simulink library "SignalGeneratorLibBtc"  (R2022b)
settings: Solver=VariableStepAuto  StartTime=0.0  StopTime=10.0  RelTol=1e-3
libraries: simulink x16, FeaturePath x6, HandyTextFile x6, RTC x6, TuneVar x1
(part 1 of 2)
settings Model: Creator=yp1048186  LastModifiedBy=kl13806
settings SolverCC: AlgebraicLoopSolver=TrustRegion
settings DebuggingCC: UnconnectedInputMsg=warning  UnconnectedOutputMsg=warning  UnconnectedLineMsg=warning  SFMachineParentedDataDiag=warning
settings ModelReferenceCC: EnableRefExpFcnMdlSchedulingChecks=on
settings RTWCC: DLArmComputeVersion=19.05

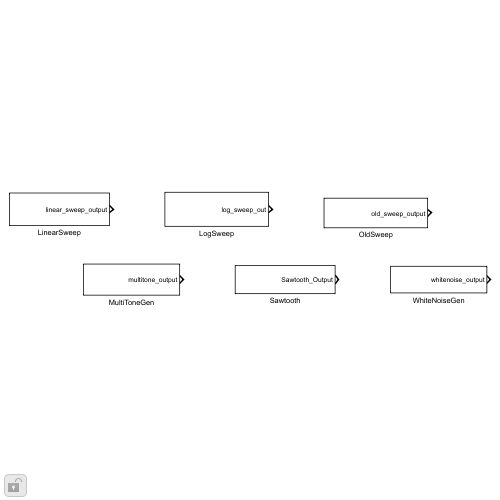
[thumbnail: Simulink's stored preview of the top-level diagram]
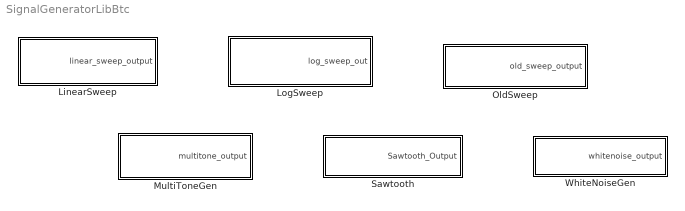
== system SignalGeneratorLibBtc ==
  LinearSweep : Subsystem  mask(Blocklib LinearSweep){Config=[], FeatureName=SignalGeneratorLinearSweep}
      mask prompts: Config "LinearSweepConfig"; FeatureName "Feature path name:"
      mask init:
      | blkh=gcbh;
      | Config=BTConfig.Assert(blkh,Config);
      | 
      | Config.Validate();
      | BTConfig.InitSetFeatureIfPresent(blkh,'FeatureName');
      mask Callback Config: BTConfig.CallbackHideIfPresent(gcbh,{'FeatureName'});
      mask TypeOptions FeatureName: FeaturePath/FeatureName
  LogSweep : Subsystem  mask(Blocklib LogSweep){Config=[], FeatureName=SignalGeneratorLogSweep}
      mask prompts: Config "LogSweepConfig"; FeatureName "Feature path name:"
      mask init:
      | blkh=gcbh;
      | Config=BTConfig.Assert(blkh,Config);
      | 
      | Config.Validate();
      | BTConfig.InitSetFeatureIfPresent(blkh,'FeatureName');
      mask Callback Config: BTConfig.CallbackHideIfPresent(gcbh,{'FeatureName'});
      mask TypeOptions FeatureName: FeaturePath/FeatureName
  MultiToneGen : Subsystem  mask(Blocklib MultiToneGen){Config=[], FeatureName=SignalGeneratorMultitone}
      mask prompts: Config "MultiToneGenConfig"; FeatureName "Feature path name:"
      mask help:
      | This block is used for generating a multi channel multi tone signal by using a sinusoid generator that supports arbirtrary frequencies by interpolating from a sine table.
      |
      | multitone_ON   :
      | Mode selection for enable/disable of multitone signal
      | 0 = Off
      | 6 = Multitone Signal
      | Example : multitone_ON =6 enables multi tone signal, multitone_ON=0 disables the multi tone signal
      |
      | multitone_channel_map   :
      | Number of tones in each channel
      | Example : multitone_channel_map = [2 3] , Indicates that there are 5 tones which needs to be mapped to 2 output channels.
      | 1st output channel has 2 tones summed up and 2nd output channel has 3 tones summed up.
      |
      | Num_Multitone_channels :
      | Indicates that there are multiple output channels ,each channel has multitone signal.
      | Example : Num_Multitone_channels=1 and multitone_channel_map =[4] means there is 1 output channel having 4 tones summed up.
      |
      | NumTones :
      | Total Number of tones
      | Example : NumTones=4 and multitone_channel_map =[4] indicates there is 1 output channel having  4 tones summed up.
      |
      | Tone_freq_Hz :
      | Vector of Frequency values in Hz for each Tone
      | Example : Tone_freq_Hz=[100 200 300]  means there are 3 tones of 100 ,200 and 300 Hz which may be assigned to 1 output channel or multiple channels
      | based on multitone_channel_map.
      | If multitone_channel_map=[1 2],this means 1st output channel will have only 100 Hz output i.e single tone signal.
      | and 2nd output channel will have 200 Hz and 300 Hz tones summed up.
      |
      | start_phase_rad :
      | Vector of Starting phase values in radians for each tone
      | Example : start_phase_rad=[0 pi/2 pi]
      |
      | ToneGains :
      | Vector of Gain values for each tone
      | Example : start_phase_rad=[0 0.25 0.5], multitone_channel_map=[3] means there is 1 output channel with 3 tones summed up and total gain observed
      | at output channel will be a sum close to 0.75
      mask init:
      | blkh=gcbh;
      | Config=BTConfig.Assert(blkh,Config);
      | 
      | Config.Validate();
      | BTConfig.InitSetFeatureIfPresent(blkh,'FeatureName');
      mask Help:
      | Configuration Parameters:
      | 
      |   multitone_ON
      |                         : mode: Vector of modes for each channel's operation
      | 						  0 = Off
      | 						  1 = Logarithmic sine sweep
      | 						  2 = Linear sine sweep
      | 						  3 = Old style sine sweep
      | 						  4 = Random noise
      | 						  5 = Sawtooth wave (Does not support sweep)
      | 						  6 = Multitone Signal
      | 						 Example : multitone_ON =6
      | 
      |   multitone_channel_map
      |                         : Number of tones in each channel
      | 						Example : multitone_channel_map = [2 3] , Indicates that there are 5 tones which needs to be mapped to 2 output channels.
      | 						1st output channel has 2 tones summed up and 2nd output channel has 3 tones summed up.
      |   Num_Multitone_channels
      |                         : Indicates that there are multiple output channels ,each channel has multitone signal.
      | 						Example : Num_Multitone_channels=1 and multitone_channel_map =[4] means there is 1 output channel having 4 tones summed up.
      |   NumTones
      |                         : Total Number of tones
      | 						Example : NumTones=4 and multitone_channel_map =[4] indicates there is 1 output channel having  4 tones summed up.
      |   Tone_freq_Hz
      |                         : Vector of Frequency values in Hz for each Tone
      | 						Example : Tone_freq_Hz=[100 200 300]  means there are 3 tones of 100 ,200 and 300 Hz which may be assigned to 1 output channel or multiple channels
      | 						based on multitone_channel_map.
      | 						If multitone_channel_map=[1 2],
      | 						this means 1st output channel will have only 100 Hz output i.e single tone signal.
      | 						and 2nd output channel will have 200 Hz and 300 Hz tones summed up.
      |   start_phase_rad
      |                         : Vector of Starting phase values in radians for each tone
      | 						Example : start_phase_rad=[0 pi/2 pi]
      |   ToneGains
      |                         : Vector of Gain values for each tone
      | 						Example : start_phase_rad=[0 0.25 0.5], multitone_channel_map=[3] means there is 1 output channel with 3 tones summed up and total gain observed
      | 						at output channel will be a sum close to 0.75
      mask Callback Config: BTConfig.CallbackHideIfPresent(gcbh,{'FeatureName'});
      mask TypeOptions FeatureName: FeaturePath/FeatureName
  OldSweep : Subsystem  mask(Blocklib OldSweep){Config=[], FeatureName=SignalGeneratorOldSweep}
      mask prompts: Config "OldSweepConfig"; FeatureName "Feature path name:"
      mask init:
      | blkh=gcbh;
      | Config=BTConfig.Assert(blkh,Config);
      | 
      | Config.Validate();
      | BTConfig.InitSetFeatureIfPresent(blkh,'FeatureName');
      mask Callback Config: BTConfig.CallbackHideIfPresent(gcbh,{'FeatureName'});
      mask TypeOptions FeatureName: FeaturePath/FeatureName
  Sawtooth : Subsystem  mask(Blocklib Sawtooth){Config=[], FeatureName=SignalGeneratorSawtooth}
      mask prompts: Config "SawtoothConfig"; FeatureName "Feature path name:"
      mask init:
      | blkh=gcbh;
      | Config=BTConfig.Assert(blkh,Config);
      | 
      | Config.Validate();
      | BTConfig.InitSetFeatureIfPresent(blkh,'FeatureName');
      mask Callback Config: BTConfig.CallbackHideIfPresent(gcbh,{'FeatureName'});
      mask TypeOptions FeatureName: FeaturePath/FeatureName
  WhiteNoiseGen : Subsystem  mask(Blocklib WhiteNoiseGen){Config=[], FeatureName=SignalGeneratorRandomNoise}
      mask prompts: Config "WhiteNoiseGenConfig"; FeatureName "Feature path name:"
      mask init:
      | blkh=gcbh;
      | Config=BTConfig.Assert(blkh,Config);
      | 
      | Config.Validate();
      | BTConfig.InitSetFeatureIfPresent(blkh,'FeatureName');
      mask Callback Config: BTConfig.CallbackHideIfPresent(gcbh,{'FeatureName'});
      mask TypeOptions FeatureName: FeaturePath/FeatureName

== system SignalGeneratorLibBtc/LinearSweep ==
  FeaturePath : FeaturePath/FeaturePath  FeatureName=SignalGeneratorLinearSweep  IsGroup=off  GroupNumber=-1  IsModule=off  TriggerInit=[615 -6 790 116]
      settings: SourceProductName=Bose Talaria
  HandyDefaultConfigFile : HandyTextFile/HandyTextFile  TemplateSource=Config  FileSuffix=Init  OpenDialogOnLoad=off  UseThisBlockName=off  AddGrandParentNamePrefix=off  TheDefaultText=|  ShowInLibBrowser=on
      | % $(FILENAME) Setup model parameters for each "Init" callback (e.g. update diagram)
      | sample_rate_in_hertz = 44100;
      | frame_size = 32;
      | sysin_channel_count = 2;
      settings: SourceProductName=Bose Talaria
  Linear Sweep Signal Generator : Subsystem
  RTC : RTC/RTC  Description=It is LinearSignal generator block  REQ_Priority=RTC_Mask.NormalPriority  RequestAtInit=off  EnableRequest=off  REQElemName1=LinearSweepOn  REQElemType1=int8  REQElemWidth1=length(Config.LinearSweepOn)  REQElemInitial1=[Config.LinearSweepOn]  REQElemName2=StartingFrequencyHz  REQElemType2=single  REQElemWidth2=length(Config.StartFreqHz)  REQElemInitial2=[Config.StartFreqHz]  REQElemName3=EndingFrequencyHz  REQElemType3=single  REQElemWidth3=length(Config.EndFreqHz)  REQElemInitial3=[Config.EndFreqHz]  REQElemName4=SweepTimeSec  REQElemType4=single  REQElemWidth4=length(Config.SweepTimeSec)  REQElemInitial4=[Config.SweepTimeSec]  REQElemName5=StartPhaseRad  REQElemType5=single  REQElemWidth5=length(Config.StartPhaseRad)  REQElemInitial5=[Config.StartPhaseRad]  REQElemType6=uint32  REQElemWidth6=1  REQElemInitial6=[]  REQElemType7=uint32  REQElemWidth7=1  REQElemInitial7=[]  REQElemType8=uint32  REQElemWidth8=1  REQElemInitial8=[]  REQElemType9=uint32  REQElemWidth9=1  REQElemInitial9=[]  REQElemType10=uint32  REQElemWidth10=1  REQElemInitial10=[]  EnableResponse=on  EnableRSP_StatusIn=off  RSPElemType1=uint32  RSPElemWidth1=1  RSPElemType2=uint32  RSPElemWidth2=1  RSPElemType3=uint32  RSPElemWidth3=1  RSPElemType4=uint32  RSPElemWidth4=1  RSPElemType5=uint32  RSPElemWidth5=1  RSPElemType6=uint32  RSPElemWidth6=1  RSPElemType7=uint32  RSPElemWidth7=1  RSPElemType8=uint32  RSPElemWidth8=1  RSPElemType9=uint32  RSPElemWidth9=1  RSPElemType10=uint32  RSPElemWidth10=1  EnableNotification=on  EnableNTF_PrepTrig=off  NTFElemType1=uint32  NTFElemWidth1=1  NTFElemType2=uint32  NTFElemWidth2=1  NTFElemType3=uint32  NTFElemWidth3=1  NTFElemType4=uint32  NTFElemWidth4=1  NTFElemType5=uint32  NTFElemWidth5=1  NTFElemType6=uint32  NTFElemWidth6=1  NTFElemType7=uint32  NTFElemWidth7=1  NTFElemType8=uint32  NTFElemWidth8=1  NTFElemType9=uint32  NTFElemWidth9=1  NTFElemType10=uint32  NTFElemWidth10=1  MaskMessageName=ConfigSet
      settings: SourceProductName=Bose Talaria
  Triggered Subsystem : Subsystem  TreatAsAtomicUnit=on
  linear_sweep_output : Outport  VectorParamsAs1DForOutWhenUnconnected=off
  wires:
  RTC/1 -> Linear Sweep Signal Generator/1(linear_sweep_ON)  "linear_sweep_mode"
  RTC/5 -> Linear Sweep Signal Generator/5(start_phase_rad)  "start_phase"
  Triggered Subsystem/1(Out1) -> RTC/1
  Linear Sweep Signal Generator/1(Linear_Sweep_Out) -> linear_sweep_output/1  "linear_sweep_output"
  RTC/4 -> Linear Sweep Signal Generator/4(sweep_time_sec)  "sweep_time"
  RTC/2 -> Linear Sweep Signal Generator/2(start_freq_Hz)  "start_freq"
  Linear Sweep Signal Generator/2(SimuliationTimeTriggerdOut1) -> Triggered Subsystem/1(In1)  "simulationtimetrigger"
  RTC/6 -> Triggered Subsystem/Trigger  "notification_trigger"
  RTC/3 -> Linear Sweep Signal Generator/3(end_freq_Hz)  "end_freq"

== system SignalGeneratorLibBtc/LogSweep ==
  FeaturePath : FeaturePath/FeaturePath  FeatureName=SignalGeneratorLogSweep  IsGroup=off  GroupNumber=-1  IsModule=off  TriggerInit=[325 -11 515 111]
      settings: SourceProductName=Bose Talaria
  HandyDefaultConfigFile : HandyTextFile/HandyTextFile  TemplateSource=Config  FileSuffix=Init  OpenDialogOnLoad=off  UseThisBlockName=off  AddGrandParentNamePrefix=off  TheDefaultText=|  ShowInLibBrowser=on
      | % $(FILENAME) Setup model parameters for each "Init" callback (e.g. update diagram)
      | sample_rate_in_hertz = 44100;
      | frame_size = 32;
      | sysin_channel_count = 2;
      settings: SourceProductName=Bose Talaria
  Log Sweep Signal Generator : Subsystem
  RTC : RTC/RTC  REQ_Priority=RTC_Mask.NormalPriority  RequestAtInit=off  EnableRequest=off  REQElemName1=LogSweepOn  REQElemType1=int8  REQElemWidth1=length(Config.LogSweepOn)  REQElemInitial1=[Config.LogSweepOn]  REQElemName2=StartingFrequencyHz  REQElemType2=single  REQElemWidth2=length(Config.StartFreqHz)  REQElemInitial2=[Config.StartFreqHz]  REQElemName3=EndingFrequencyHz  REQElemType3=single  REQElemWidth3=length(Config.EndFreqHz)  REQElemInitial3=[Config.EndFreqHz]  REQElemName4=SweepTimeSec  REQElemType4=single  REQElemWidth4=length(Config.SweepTimeSec)  REQElemInitial4=[Config.SweepTimeSec]  REQElemName5=StartPhaseRad  REQElemType5=single  REQElemWidth5=length(Config.StartPhaseRad)  REQElemInitial5=[Config.StartPhaseRad]  REQElemType6=uint32  REQElemWidth6=1  REQElemInitial6=[]  REQElemType7=uint32  REQElemWidth7=1  REQElemInitial7=[]  REQElemType8=uint32  REQElemWidth8=1  REQElemInitial8=[]  REQElemType9=uint32  REQElemWidth9=1  REQElemInitial9=[]  REQElemType10=uint32  REQElemWidth10=1  REQElemInitial10=[]  EnableResponse=on  EnableRSP_StatusIn=off  RSPElemType1=uint32  RSPElemWidth1=1  RSPElemType2=uint32  RSPElemWidth2=1  RSPElemType3=uint32  RSPElemWidth3=1  RSPElemType4=uint32  RSPElemWidth4=1  RSPElemType5=uint32  RSPElemWidth5=1  RSPElemType6=uint32  RSPElemWidth6=1  RSPElemType7=uint32  RSPElemWidth7=1  RSPElemType8=uint32  RSPElemWidth8=1  RSPElemType9=uint32  RSPElemWidth9=1  RSPElemType10=uint32  RSPElemWidth10=1  EnableNotification=on  EnableNTF_PrepTrig=off  NTFElemType1=uint32  NTFElemWidth1=1  NTFElemType2=uint32  NTFElemWidth2=1  NTFElemType3=uint32  NTFElemWidth3=1  NTFElemType4=uint32  NTFElemWidth4=1  NTFElemType5=uint32  NTFElemWidth5=1  NTFElemType6=uint32  NTFElemWidth6=1  NTFElemType7=uint32  NTFElemWidth7=1  NTFElemType8=uint32  NTFElemWidth8=1  NTFElemType9=uint32  NTFElemWidth9=1  NTFElemType10=uint32  NTFElemWidth10=1  MaskMessageName=ConfigSet
      settings: SourceProductName=Bose Talaria
  TriggeredSubsystem : Subsystem  TreatAsAtomicUnit=on
  log_sweep_out : Outport  VectorParamsAs1DForOutWhenUnconnected=off
  wires:
  Log Sweep Signal Generator/1(Log_Sweep_Out) -> log_sweep_out/1  "log_sweep_out"
  Log Sweep Signal Generator/2(SimuliationTimeTriggerdOut1) -> TriggeredSubsystem/1(In1)  "simulationtimetrigger"
  RTC/4 -> Log Sweep Signal Generator/4(sweep_time_sec)  "sweep_time"
  RTC/6 -> TriggeredSubsystem/Trigger  "notification_trigger"
  TriggeredSubsystem/1(Out1) -> RTC/1
  RTC/5 -> Log Sweep Signal Generator/5(start_phase_rad)  "start_phase"
  RTC/3 -> Log Sweep Signal Generator/3(end_freq_Hz)  "end_freq"
  RTC/2 -> Log Sweep Signal Generator/2(start_freq_Hz)  "start_freq"
  RTC/1 -> Log Sweep Signal Generator/1(log_sweep_ON)  "log_sweep_mode"

== system SignalGeneratorLibBtc/MultiToneGen ==
  FeaturePath : FeaturePath/FeaturePath  FeatureName=SignalGeneratorMultitone  IsGroup=off  GroupNumber=-1  IsModule=off  TriggerInit=[1660 324 1835 466]
      settings: SourceProductName=Bose Talaria
  HandyDefaultConfigFile : HandyTextFile/HandyTextFile  TemplateSource=Config  FileSuffix=Init  OpenDialogOnLoad=off  UseThisBlockName=off  AddGrandParentNamePrefix=off  TheDefaultText=|  ShowInLibBrowser=on
      | % $(FILENAME) Setup model parameters for each "Init" callback (e.g. update diagram)
      | sample_rate_in_hertz = 44100;
      | frame_size = 32;
      | sysin_channel_count = 2;
      settings: SourceProductName=Bose Talaria
  Multitone Signal Generator : Subsystem
  RTC : RTC/RTC  REQ_Priority=RTC_Mask.NormalPriority  RequestAtInit=off  EnableRequest=off  REQElemName1=MultitoneModeOn  REQElemType1=int8  REQElemWidth1=length(Config.MultitoneOn)  REQElemInitial1=[Config.MultitoneOn]  REQElemName2=ToneFreqHz  REQElemType2=single  REQElemWidth2=length(Config.ToneFreqHz)  REQElemInitial2=[Config.ToneFreqHz]  REQElemName3=StartPhaseRad  REQElemType3=single  REQElemWidth3=length(Config.StartPhaseRad)  REQElemInitial3=[Config.StartPhaseRad]  REQElemName4=ToneGain  REQElemType4=single  REQElemWidth4=length(Config.ToneGains)  REQElemInitial4=[Config.ToneGains]  REQElemName5=MultitoneChannelMapSequence  REQElemType5=uint8  REQElemWidth5=length(Config.MultitoneChannelMap)  REQElemInitial5=[Config.MultitoneChannelMap]  REQElemType6=uint32  REQElemWidth6=1  REQElemInitial6=[]  REQElemType7=uint32  REQElemWidth7=1  REQElemInitial7=[]  REQElemType8=uint32  REQElemWidth8=1  REQElemInitial8=[]  REQElemType9=uint32  REQElemWidth9=1  REQElemInitial9=[]  REQElemType10=uint32  REQElemWidth10=1  REQElemInitial10=[]  EnableResponse=on  EnableRSP_StatusIn=off  RSPElemType1=uint32  RSPElemWidth1=1  RSPElemType2=uint32  RSPElemWidth2=1  RSPElemType3=uint32  RSPElemWidth3=1  RSPElemType4=uint32  RSPElemWidth4=1  RSPElemType5=uint32  RSPElemWidth5=1  RSPElemType6=uint32  RSPElemWidth6=1  RSPElemType7=uint32  RSPElemWidth7=1  RSPElemType8=uint32  RSPElemWidth8=1  RSPElemType9=uint32  RSPElemWidth9=1  RSPElemType10=uint32  RSPElemWidth10=1  EnableNotification=off  EnableNTF_PrepTrig=off  NTFElemType1=uint32  NTFElemWidth1=1  NTFElemType2=uint32  NTFElemWidth2=1  NTFElemType3=uint32  NTFElemWidth3=1  NTFElemType4=uint32  NTFElemWidth4=1  NTFElemType5=uint32  NTFElemWidth5=1  NTFElemType6=uint32  NTFElemWidth6=1  NTFElemType7=uint32  NTFElemWidth7=1  NTFElemType8=uint32  NTFElemWidth8=1  NTFElemType9=uint32  NTFElemWidth9=1  NTFElemType10=uint32  NTFElemWidth10=1  MaskMessageName=ConfigSet
      settings: SourceProductName=Bose Talaria
  multitone_output : Outport  VectorParamsAs1DForOutWhenUnconnected=off
  wires:
  RTC/5 -> Multitone Signal Generator/5(ChannelMap)  "notification_trigger"
  Multitone Signal Generator/1(Multitone_Out) -> multitone_output/1  "multitone_output"
  RTC/2 -> Multitone Signal Generator/2(start_freq_Hz)
  RTC/3 -> Multitone Signal Generator/3(start_phase_rad)  "start_phase"
  RTC/4 -> Multitone Signal Generator/4(ToneGains)
  RTC/1 -> Multitone Signal Generator/1(multitone_ON)  "multitone_mode"

== system SignalGeneratorLibBtc/OldSweep ==
  FeaturePath : FeaturePath/FeaturePath  FeatureName=SignalGeneratorOldSweep  IsGroup=off  GroupNumber=-1  IsModule=off  TriggerInit=[380 -1 565 131]
      settings: SourceProductName=Bose Talaria
  HandyDefaultConfigFile : HandyTextFile/HandyTextFile  TemplateSource=Config  FileSuffix=Init  OpenDialogOnLoad=off  UseThisBlockName=off  AddGrandParentNamePrefix=off  TheDefaultText=|  ShowInLibBrowser=on
      | % $(FILENAME) Setup model parameters for each "Init" callback (e.g. update diagram)
      | sample_rate_in_hertz = 44100;
      | frame_size = 32;
      | sysin_channel_count = 2;
      settings: SourceProductName=Bose Talaria
  Old Sweep Signal Generator : Subsystem
  RTC : RTC/RTC  REQ_Priority=RTC_Mask.NormalPriority  RequestAtInit=off  EnableRequest=off  REQElemName1=OldSweepOn  REQElemType1=int8  REQElemWidth1=length(Config.OldSweepOn)  REQElemInitial1=[Config.OldSweepOn]  REQElemName2=StartingFrequencyHz  REQElemType2=single  REQElemWidth2=length(Config.StartFreqHz)  REQElemInitial2=[Config.StartFreqHz]  REQElemName3=EndingFrequencyHz  REQElemType3=single  REQElemWidth3=length(Config.EndFreqHz)  REQElemInitial3=[Config.EndFreqHz]  REQElemName4=Steps  REQElemType4=int32  REQElemWidth4=length(Config.Steps)  REQElemInitial4=[Config.Steps]  REQElemName5=StartPhaseRad  REQElemType5=single  REQElemWidth5=length(Config.StartPhaseRad)  REQElemInitial5=[Config.StartPhaseRad]  REQElemName6=CyclesPerStep  REQElemType6=int32  REQElemWidth6=length(Config.CyclesPerStepc)  REQElemInitial6=[Config.CyclesPerStepc]  REQElemType7=uint32  REQElemWidth7=1  REQElemInitial7=[]  REQElemType8=uint32  REQElemWidth8=1  REQElemInitial8=[]  REQElemType9=uint32  REQElemWidth9=1  REQElemInitial9=[]  REQElemType10=uint32  REQElemWidth10=1  REQElemInitial10=[]  EnableResponse=on  EnableRSP_StatusIn=off  RSPElemType1=uint32  RSPElemWidth1=1  RSPElemType2=uint32  RSPElemWidth2=1  RSPElemType3=uint32  RSPElemWidth3=1  RSPElemType4=uint32  RSPElemWidth4=1  RSPElemType5=uint32  RSPElemWidth5=1  RSPElemType6=uint32  RSPElemWidth6=1  RSPElemType7=uint32  RSPElemWidth7=1  RSPElemType8=uint32  RSPElemWidth8=1  RSPElemType9=uint32  RSPElemWidth9=1  RSPElemType10=uint32  RSPElemWidth10=1  EnableNotification=on  EnableNTF_PrepTrig=off  NTFElemType1=uint32  NTFElemWidth1=1  NTFElemType2=uint32  NTFElemWidth2=1  NTFElemType3=uint32  NTFElemWidth3=1  NTFElemType4=uint32  NTFElemWidth4=1  NTFElemType5=uint32  NTFElemWidth5=1  NTFElemType6=uint32  NTFElemWidth6=1  NTFElemType7=uint32  NTFElemWidth7=1  NTFElemType8=uint32  NTFElemWidth8=1  NTFElemType9=uint32  NTFElemWidth9=1  NTFElemType10=uint32  NTFElemWidth10=1  MaskMessageName=ConfigSet
      settings: SourceProductName=Bose Talaria
  Triggered Subsystem : Subsystem  TreatAsAtomicUnit=on
  old_sweep_output : Outport  VectorParamsAs1DForOutWhenUnconnected=off
  wires:
  Old Sweep Signal Generator/1(Old_sweep_Out) -> old_sweep_output/1  "old_sweep_output"
  RTC/5 -> Old Sweep Signal Generator/5(start_phase_rad)  "start_phase"
  RTC/7 -> Triggered Subsystem/Trigger  "notification_trigger"
  RTC/1 -> Old Sweep Signal Generator/1(old_sweep_ON)  "old_sweep_mode"
  RTC/6 -> Old Sweep Signal Generator/6(cycles_per_step)  "cycels_per_step"
  RTC/4 -> Old Sweep Signal Generator/4(steps)  "steps"
  Old Sweep Signal Generator/2(SimuliationTimeTriggerdOut1) -> Triggered Subsystem/1(In1)
  RTC/2 -> Old Sweep Signal Generator/2(start_freq_Hz)  "start_freq"
  Triggered Subsystem/1(Out1) -> RTC/1
  RTC/3 -> Old Sweep Signal Generator/3(end_freq_Hz)  "end_freq"

== system SignalGeneratorLibBtc/Sawtooth ==
  FeaturePath : FeaturePath/FeaturePath  FeatureName=SignalGeneratorSawtooth  IsGroup=off  GroupNumber=-1  IsModule=off  TriggerInit=[290 -216 460 -109]
      settings: SourceProductName=Bose Talaria
  HandyDefaultConfigFile : HandyTextFile/HandyTextFile  TemplateSource=Config  FileSuffix=Init  OpenDialogOnLoad=off  UseThisBlockName=off  AddGrandParentNamePrefix=off  TheDefaultText=|  ShowInLibBrowser=on
      | % $(FILENAME) Setup model parameters for each "Init" callback (e.g. update diagram)
      | sample_rate_in_hertz = 44100;
      | frame_size = 32;
      | sysin_channel_count = 2;
      settings: SourceProductName=Bose Talaria
  RTC : RTC/RTC  REQ_Priority=RTC_Mask.NormalPriority  RequestAtInit=off  EnableRequest=off  REQElemName1=SawtoothModeOn  REQElemType1=int8  REQElemWidth1=length(Config.SawtoothModeOn)  REQElemInitial1=[Config.SawtoothModeOn]  REQElemName2=StartingPhase  REQElemType2=single  REQElemWidth2=length(Config.StartPhaseRad)  REQElemInitial2=[Config.StartPhaseRad]  REQElemName3=StartingFrequency  REQElemType3=single  REQElemWidth3=length(Config.StartFreqHz)  REQElemInitial3=[Config.StartFreqHz]  REQElemType4=uint32  REQElemWidth4=1  REQElemInitial4=[]  REQElemType5=uint32  REQElemWidth5=1  REQElemInitial5=[]  REQElemType6=uint32  REQElemWidth6=1  REQElemInitial6=[]  REQElemType7=uint32  REQElemWidth7=1  REQElemInitial7=[]  REQElemType8=uint32  REQElemWidth8=1  REQElemInitial8=[]  REQElemType9=uint32  REQElemWidth9=1  REQElemInitial9=[]  REQElemType10=uint32  REQElemWidth10=1  REQElemInitial10=[]  EnableResponse=on  EnableRSP_StatusIn=off  RSPElemType1=uint32  RSPElemWidth1=1  RSPElemType2=uint32  RSPElemWidth2=1  RSPElemType3=uint32  RSPElemWidth3=1  RSPElemType4=uint32  RSPElemWidth4=1  RSPElemType5=uint32  RSPElemWidth5=1  RSPElemType6=uint32  RSPElemWidth6=1  RSPElemType7=uint32  RSPElemWidth7=1  RSPElemType8=uint32  RSPElemWidth8=1  RSPElemType9=uint32  RSPElemWidth9=1  RSPElemType10=uint32  RSPElemWidth10=1  EnableNotification=on  EnableNTF_PrepTrig=off  NTFElemType1=uint32  NTFElemWidth1=1  NTFElemType2=uint32  NTFElemWidth2=1  NTFElemType3=uint32  NTFElemWidth3=1  NTFElemType4=uint32  NTFElemWidth4=1  NTFElemType5=uint32  NTFElemWidth5=1  NTFElemType6=uint32  NTFElemWidth6=1  NTFElemType7=uint32  NTFElemWidth7=1  NTFElemType8=uint32  NTFElemWidth8=1  NTFElemType9=uint32  NTFElemWidth9=1  NTFElemType10=uint32  NTFElemWidth10=1  MaskMessageName=ConfigSet
      settings: SourceProductName=Bose Talaria
  SawtoothGenSubsystem : Subsystem  TreatAsAtomicUnit=on
  Transpose : Math  Operator=transpose  SignedPower=on
  Transpose1 : Math  Operator=transpose  SignedPower=on
  Transpose2 : Math  Operator=transpose  SignedPower=on
  Triggered Subsystem : Subsystem  TreatAsAtomicUnit=on
  TuneTOP_time : TuneVar/TuneTOP  TriggerInit=[35 387 140 423]  TopName=tuneTop_time  TuneName=tuneTop_time  DataType=single  TunabilityNumber=1  MinValue=[]  MaxValue=[]  BankNumber=0  PreOverlay=false  PostOverlay=false  UseSameName=on  MaskValue=Config.DefaultTuneTopTime
      settings: SourceProductName=Bose Talaria
  Sawtooth_Output : Outport  VectorParamsAs1DForOutWhenUnconnected=off
  wires:
  RTC/3 -> Transpose2/1
  RTC/2 -> Transpose1/1
  RTC/1 -> Transpose/1
  Triggered Subsystem/1(Out1) -> RTC/1
  SawtoothGenSubsystem/2(Out2) -> Triggered Subsystem/1(In1)
  RTC/4 -> Triggered Subsystem/Trigger
  Transpose2/1 -> SawtoothGenSubsystem/3(startfreq)
  SawtoothGenSubsystem/1(sawtooth_output) -> Sawtooth_Output/1
  Transpose1/1 -> SawtoothGenSubsystem/2(start_phase_In)
  Transpose/1 -> SawtoothGenSubsystem/1(mode_In1)
  TuneTOP_time/1 -> SawtoothGenSubsystem/4(tuneable_time_In4)

== system SignalGeneratorLibBtc/WhiteNoiseGen ==
  FeaturePath : FeaturePath/FeaturePath  FeatureName=SignalGeneratorRandomNoise  IsGroup=off  GroupNumber=-1  IsModule=off  TriggerInit=[295 -196 535 -84]
      settings: SourceProductName=Bose Talaria
  ForEachSubsystem : Subsystem  TreatAsAtomicUnit=on
  HandyDefaultConfigFile : HandyTextFile/HandyTextFile  TemplateSource=Config  FileSuffix=Init  OpenDialogOnLoad=off  UseThisBlockName=off  AddGrandParentNamePrefix=off  TheDefaultText=|  ShowInLibBrowser=on
      | % $(FILENAME) Setup model parameters for each "Init" callback (e.g. update diagram)
      | sample_rate_in_hertz = 44100;
      | frame_size = 32;
      | sysin_channel_count = 2;
      settings: SourceProductName=Bose Talaria
  RTC : RTC/RTC  REQ_Priority=RTC_Mask.NormalPriority  RequestAtInit=off  EnableRequest=off  REQElemName1=WhiteNoiseModeOn  REQElemType1=int8  REQElemWidth1=length(Config.RandomNoiseOn)  REQElemInitial1=[]  REQElemName2=RandomNoise  REQElemType2=single  REQElemWidth2=length(Config.RandomNoise)  REQElemInitial2=[]  REQElemType3=uint32  REQElemWidth3=1  REQElemInitial3=[]  REQElemType4=uint32  REQElemWidth4=1  REQElemInitial4=[]  REQElemType5=uint32  REQElemWidth5=1  REQElemInitial5=[]  REQElemType6=uint32  REQElemWidth6=1  REQElemInitial6=[]  REQElemType7=uint32  REQElemWidth7=1  REQElemInitial7=[]  REQElemType8=uint32  REQElemWidth8=1  REQElemInitial8=[]  REQElemType9=uint32  REQElemWidth9=1  REQElemInitial9=[]  REQElemType10=uint32  REQElemWidth10=1  REQElemInitial10=[]  EnableResponse=on  EnableRSP_StatusIn=off  RSPElemType1=uint32  RSPElemWidth1=1  RSPElemType2=uint32  RSPElemWidth2=1  RSPElemType3=uint32  RSPElemWidth3=1  RSPElemType4=uint32  RSPElemWidth4=1  RSPElemType5=uint32  RSPElemWidth5=1  RSPElemType6=uint32  RSPElemWidth6=1  RSPElemType7=uint32  RSPElemWidth7=1  RSPElemType8=uint32  RSPElemWidth8=1  RSPElemType9=uint32  RSPElemWidth9=1  RSPElemType10=uint32  RSPElemWidth10=1  EnableNotification=on  EnableNTF_PrepTrig=off  NTFElemType1=uint32  NTFElemWidth1=1  NTFElemType2=uint32  NTFElemWidth2=1  NTFElemType3=uint32  NTFElemWidth3=1  NTFElemType4=uint32  NTFElemWidth4=1  NTFElemType5=uint32  NTFElemWidth5=1  NTFElemType6=uint32  NTFElemWidth6=1  NTFElemType7=uint32  NTFElemWidth7=1  NTFElemType8=uint32  NTFElemWidth8=1  NTFElemType9=uint32  NTFElemWidth9=1  NTFElemType10=uint32  NTFElemWidth10=1  MaskMessageName=ConfigSet
      settings: SourceProductName=Bose Talaria
  Transpose : Math  Operator=transpose  SignedPower=on
  Transpose6 : Math  Operator=transpose  SignedPower=on
  Triggered Subsystem : Subsystem  TreatAsAtomicUnit=on
  whitenoise_output : Outport  VectorParamsAs1DForOutWhenUnconnected=off
  wires:
  Triggered Subsystem/1(Out1) -> RTC/1
  RTC/3 -> Triggered Subsystem/Trigger  "notification_trigger"
  ForEachSubsystem/2(SimuliationTimeTriggerdOut1) -> Triggered Subsystem/1(In1)
  Transpose/1 -> ForEachSubsystem/1(mode_In1)
  Transpose6/1 -> ForEachSubsystem/2(random_noise_In)
  RTC/2 -> Transpose6/1  "random_noise"
  ForEachSubsystem/1(noise_outpupt) -> whitenoise_output/1
  RTC/1 -> Transpose/1  "randomnoise_mode"

== system SignalGeneratorLibBtc/LinearSweep/Linear Sweep Signal Generator ==
  linear_sweep_ON : Inport
  start_freq_Hz : Inport  Port=2
  end_freq_Hz : Inport  Port=3
  sweep_time_sec : Inport  Port=4
  start_phase_rad : Inport  Port=5
  Linear Sweep Engine : Subsystem  TreatAsAtomicUnit=on
  SimulationTimeTriggered_Subsystem : Subsystem
  Linear_Sweep_Out : Outport  VectorParamsAs1DForOutWhenUnconnected=off
  SimuliationTimeTriggerdOut1 : Outport  Port=2  VectorParamsAs1DForOutWhenUnconnected=off
  wires:
  SimulationTimeTriggered_Subsystem/1(SimuliationTimeTriggerdOut1) -> SimuliationTimeTriggerdOut1/1
  start_phase_rad/1 -> Linear Sweep Engine/5(start_phase_In)
  sweep_time_sec/1 -> Linear Sweep Engine/4(sweep_time_In)
  end_freq_Hz/1 -> Linear Sweep Engine/3(end_freq_In)
  start_freq_Hz/1 -> Linear Sweep Engine/2(start_freq_In)
  linear_sweep_ON/1 -> Linear Sweep Engine/1(linear_sweep_ON)
  Linear Sweep Engine/1(Linear_Sweep_Out) -> Linear_Sweep_Out/1

== system SignalGeneratorLibBtc/LinearSweep/Triggered Subsystem ==
  In1 : Inport
  Trigger : TriggerPort  TriggerType=function-call  VariantControl=Variant
  Out1 : Outport  VectorParamsAs1DForOutWhenUnconnected=off
  wires:
  In1/1 -> Out1/1

== system SignalGeneratorLibBtc/LogSweep/Log Sweep Signal Generator ==
  log_sweep_ON : Inport
  start_freq_Hz : Inport  Port=2
  end_freq_Hz : Inport  Port=3
  sweep_time_sec : Inport  Port=4
  start_phase_rad : Inport  Port=5
  Log Sweep Engine : Subsystem  TreatAsAtomicUnit=on
  SimulationTimeTriggered_Subsystem : Subsystem
  Log_Sweep_Out : Outport  VectorParamsAs1DForOutWhenUnconnected=off
  SimuliationTimeTriggerdOut1 : Outport  Port=2  VectorParamsAs1DForOutWhenUnconnected=off
  wires:
  SimulationTimeTriggered_Subsystem/1(SimuliationTimeTriggerdOut1) -> SimuliationTimeTriggerdOut1/1
  start_phase_rad/1 -> Log Sweep Engine/5(start_phase_In)  "start_phase"
  sweep_time_sec/1 -> Log Sweep Engine/4(sweep_time_In)  "sweep_time"
  end_freq_Hz/1 -> Log Sweep Engine/3(end_freq_In)  "end_freq"
  start_freq_Hz/1 -> Log Sweep Engine/2(start_freq_In)  "start_freq"
  log_sweep_ON/1 -> Log Sweep Engine/1(log_sweep_ON)  "log_sweep_mode"
  Log Sweep Engine/1(Log_Sweep_Out) -> Log_Sweep_Out/1  "log_sweep_output"

== system SignalGeneratorLibBtc/LogSweep/TriggeredSubsystem ==
  In1 : Inport
  Trigger : TriggerPort  TriggerType=function-call  VariantControl=Variant
  Out1 : Outport  VectorParamsAs1DForOutWhenUnconnected=off
  wires:
  In1/1 -> Out1/1

== system SignalGeneratorLibBtc/MultiToneGen/Multitone Signal Generator ==
  multitone_ON : Inport
  start_freq_Hz : Inport  Port=2
  start_phase_rad : Inport  Port=3
  ToneGains : Inport  Port=4
  ChannelMap : Inport  Port=5
  Multitone Engine : Subsystem  TreatAsAtomicUnit=on
  Multitone_Out : Outport  VectorParamsAs1DForOutWhenUnconnected=off
  wires:
  ChannelMap/1 -> Multitone Engine/5(ChannelMap)
  Multitone Engine/1(Multitone_Out) -> Multitone_Out/1
  start_phase_rad/1 -> Multitone Engine/3(start_phase_In)  "start_phase"
  start_freq_Hz/1 -> Multitone Engine/2(start_freq_In)  "start_freq"
  multitone_ON/1 -> Multitone Engine/1(multitone_ON)  "multitone_mode"
  ToneGains/1 -> Multitone Engine/4(ToneGains)

== system SignalGeneratorLibBtc/OldSweep/Old Sweep Signal Generator ==
  old_sweep_ON : Inport
  start_freq_Hz : Inport  Port=2
  end_freq_Hz : Inport  Port=3
  steps : Inport  Port=4
  start_phase_rad : Inport  Port=5
  cycles_per_step : Inport  Port=6
  Old Sweep Engine : Subsystem  TreatAsAtomicUnit=on
  SimulationTimeTriggered_Subsystem : Subsystem
  Old_sweep_Out : Outport  VectorParamsAs1DForOutWhenUnconnected=off
  SimuliationTimeTriggerdOut1 : Outport  Port=2  VectorParamsAs1DForOutWhenUnconnected=off
  wires:
  SimulationTimeTriggered_Subsystem/1(SimuliationTimeTriggerdOut1) -> SimuliationTimeTriggerdOut1/1
  cycles_per_step/1 -> Old Sweep Engine/6(cycles_per_step)
  start_phase_rad/1 -> Old Sweep Engine/5(start_phase_In)
  steps/1 -> Old Sweep Engine/4(steps_In)
  end_freq_Hz/1 -> Old Sweep Engine/3(end_freq_In)
  start_freq_Hz/1 -> Old Sweep Engine/2(start_freq_In)
  old_sweep_ON/1 -> Old Sweep Engine/1(old_sweep_ON)
  Old Sweep Engine/1(Old_Sweep_Out) -> Old_sweep_Out/1

== system SignalGeneratorLibBtc/OldSweep/Triggered Subsystem ==
  In1 : Inport
  Trigger : TriggerPort  TriggerType=function-call  VariantControl=Variant
  Out1 : Outport  VectorParamsAs1DForOutWhenUnconnected=off
  wires:
  In1/1 -> Out1/1

== system SignalGeneratorLibBtc/Sawtooth/SawtoothGenSubsystem ==
  mode_In1 : Inport
  start_phase_In : Inport  Port=2
  startfreq : Inport  Port=3
  tuneable_time_In4 : Inport  Port=4
  SimulationTimeTriggered_Subsystem : Subsystem
  Subsystem : Subsystem
  Terminator : Terminator
  sawtooth_output : Outport  VectorParamsAs1DForOutWhenUnconnected=off
  Out2 : Outport  Port=2  VectorParamsAs1DForOutWhenUnconnected=off
  wires:
  mode_In1/1 -> Subsystem/1(In1)
  startfreq/1 -> Subsystem/2(In2)
  start_phase_In/1 -> Subsystem/3(In3)
  SimulationTimeTriggered_Subsystem/1(SimuliationTimeTriggerdOut1) -> Out2/1
  tuneable_time_In4/1 -> Terminator/1
  Subsystem/1(sawtooth_output) -> sawtooth_output/1

== system SignalGeneratorLibBtc/Sawtooth/Triggered Subsystem ==
  In1 : Inport
  Trigger : TriggerPort  TriggerType=function-call  VariantControl=Variant
  Out1 : Outport  VectorParamsAs1DForOutWhenUnconnected=off
  wires:
  In1/1 -> Out1/1

== system SignalGeneratorLibBtc/WhiteNoiseGen/ForEachSubsystem ==
  mode_In1 : Inport
  random_noise_In : Inport  Port=2
  Disable_Noise : Subsystem  TreatAsAtomicUnit=on
  If_mode_selection : If  IfExpression=(u1==4)
  Merge : Merge
  SigGen_Noise : Subsystem  TreatAsAtomicUnit=on
  SimulationTimeTriggered_Subsystem : Subsystem
  noise_outpupt : Outport  VectorParamsAs1DForOutWhenUnconnected=off
  SimuliationTimeTriggerdOut1 : Outport  Port=2  VectorParamsAs1DForOutWhenUnconnected=off
  wires:
  SimulationTimeTriggered_Subsystem/1(SimuliationTimeTriggerdOut1) -> SimuliationTimeTriggerdOut1/1
  mode_In1/1 -> If_mode_selection/1  "random_noise_mode"
  If_mode_selection/1 -> SigGen_Noise/Action
  random_noise_In/1 -> SigGen_Noise/1(randomnoise)  "random_noise"
  SigGen_Noise/1(noiseOut1) -> Merge/1  "noise_output"
  If_mode_selection/2 -> Disable_Noise/Action
  Disable_Noise/1(Output) -> Merge/2  "Disable_noise_output"
  Merge/1 -> noise_outpupt/1

== system SignalGeneratorLibBtc/WhiteNoiseGen/Triggered Subsystem ==
  In1 : Inport
  Trigger : TriggerPort  TriggerType=function-call  VariantControl=Variant
  Out1 : Outport  VectorParamsAs1DForOutWhenUnconnected=off
  wires:
  In1/1 -> Out1/1

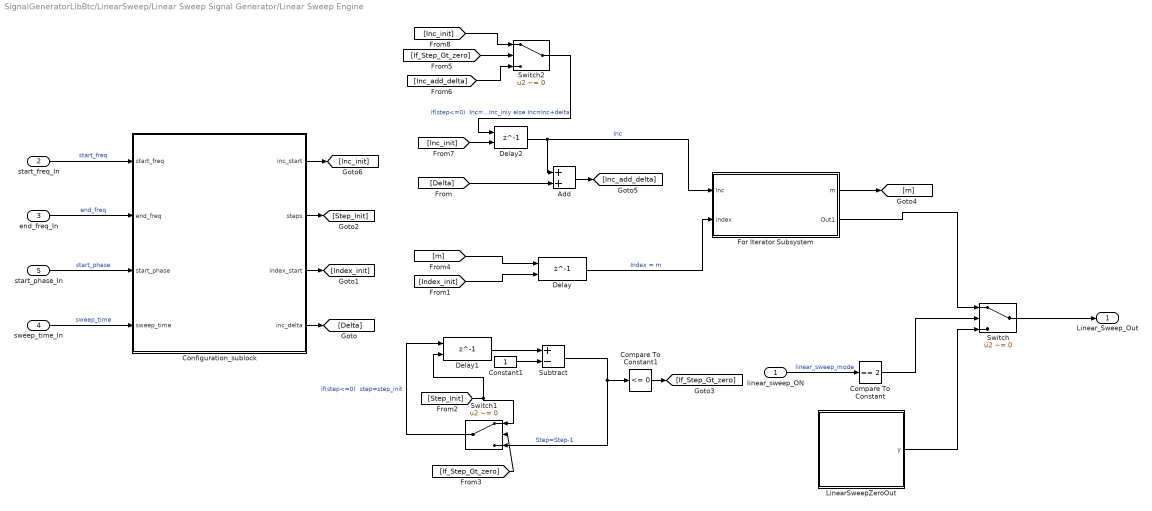
== system SignalGeneratorLibBtc/LinearSweep/Linear Sweep Signal Generator/Linear Sweep Engine ==
  linear_sweep_ON : Inport
  start_freq_In : Inport  Port=2
  end_freq_In : Inport  Port=3
  sweep_time_In : Inport  Port=4
  start_phase_In : Inport  Port=5
  Add : Sum
  Compare To Constant : simulink/Logic and Bit Operations/Compare To Constant  relop===  const=2  OutDataTypeStr=boolean
  Compare To Constant1 : simulink/Logic and Bit Operations/Compare To Constant  relop=<=  const=0  OutDataTypeStr=boolean
  Configuration_sublock : Subsystem
  Constant1 : Constant  OutDataTypeStr=single
  Delay : Delay  DelayLength=1  InitialConditionSource=Input port
      settings: InputPortMap=u0,p4
  Delay1 : Delay  DelayLength=1  InitialConditionSource=Input port
      settings: InputPortMap=u0,p4
  Delay2 : Delay  DelayLength=1  InitialConditionSource=Input port
      settings: InputPortMap=u0,p4
  For Iterator Subsystem : Subsystem  TreatAsAtomicUnit=on
  LinearSweepZeroOut : MATLAB Function  TreatAsAtomicUnit=on  mask{Nch=Config.NumChannel, frameSize_samples=Config.FrameSizeSamples}
  Subtract : Sum  Inputs=+-
  Switch : Switch  Criteria=u2 ~= 0  SaturateOnIntegerOverflow=off  InputSameDT=off
  Switch1 : Switch  Criteria=u2 ~= 0  SaturateOnIntegerOverflow=off  InputSameDT=off
  Switch2 : Switch  Criteria=u2 ~= 0  SaturateOnIntegerOverflow=off  InputSameDT=off
  Linear_Sweep_Out : Outport  VectorParamsAs1DForOutWhenUnconnected=off
  wires:
  LinearSweepZeroOut/1(y) -> Switch/3
  Delay2/1 -> Add/1, For Iterator Subsystem/1("Inc ")  "Inc"
  Configuration_sublock/4(inc_delta) -> [Delta]
  [Delta] -> Add/2
  [m] -> Delay/1
  Switch1/1 -> Delay1/1  "if(step<=0)  step=step_init"
  [Inc_add_delta] -> Switch2/3
  Delay1/1 -> Subtract/1
  [If_Step_Gt_zero] -> Switch2/2
  [Step_Init] -> Delay1/2, Switch1/1
  start_phase_In/1 -> Configuration_sublock/3(start_phase)  "start_phase"
  Compare To Constant1/1 -> [If_Step_Gt_zero]
  Add/1 -> [Inc_add_delta]
  [Inc_init] -> Delay2/2
  Constant1/1 -> Subtract/2
  Configuration_sublock/1(inc_start) -> [Inc_init]
  For Iterator Subsystem/2(Out1) -> Switch/1
  Compare To Constant/1 -> Switch/2
  [Inc_init] -> Switch2/1
  Switch2/1 -> Delay2/1  "if(step<=0)  Inc=Inc_iniy else Inc=Inc+delta"
  [If_Step_Gt_zero] -> Switch1/2
  Subtract/1 -> Switch1/3, Compare To Constant1/1  "Step=Step-1"
  Delay/1 -> For Iterator Subsystem/2(index)  "Index = m"
  start_freq_In/1 -> Configuration_sublock/1(start_freq)  "start_freq"
  For Iterator Subsystem/1(m) -> [m]
  linear_sweep_ON/1 -> Compare To Constant/1  "linear_sweep_mode"
  Configuration_sublock/2(steps) -> [Step_Init]
  [Index_init] -> Delay/2
  Switch/1 -> Linear_Sweep_Out/1
  end_freq_In/1 -> Configuration_sublock/2(end_freq)  "end_freq"
  sweep_time_In/1 -> Configuration_sublock/4("sweep_time ")  "sweep_time"
  Configuration_sublock/3(index_start) -> [Index_init]

== system SignalGeneratorLibBtc/LinearSweep/Linear Sweep Signal Generator/SimulationTimeTriggered_Subsystem ==
  Constant : Constant
  Digital Clock : DigitalClock  SampleTime=-1
  Equal : RelationalOperator  Operator===  OutDataTypeStr=boolean  RndMeth=Simplest  InputSameDT=off
  SimuliationTimeTriggerdOut1 : Outport  VectorParamsAs1DForOutWhenUnconnected=off
  wires:
  Equal/1 -> SimuliationTimeTriggerdOut1/1
  Constant/1 -> Equal/1
  Digital Clock/1 -> Equal/2

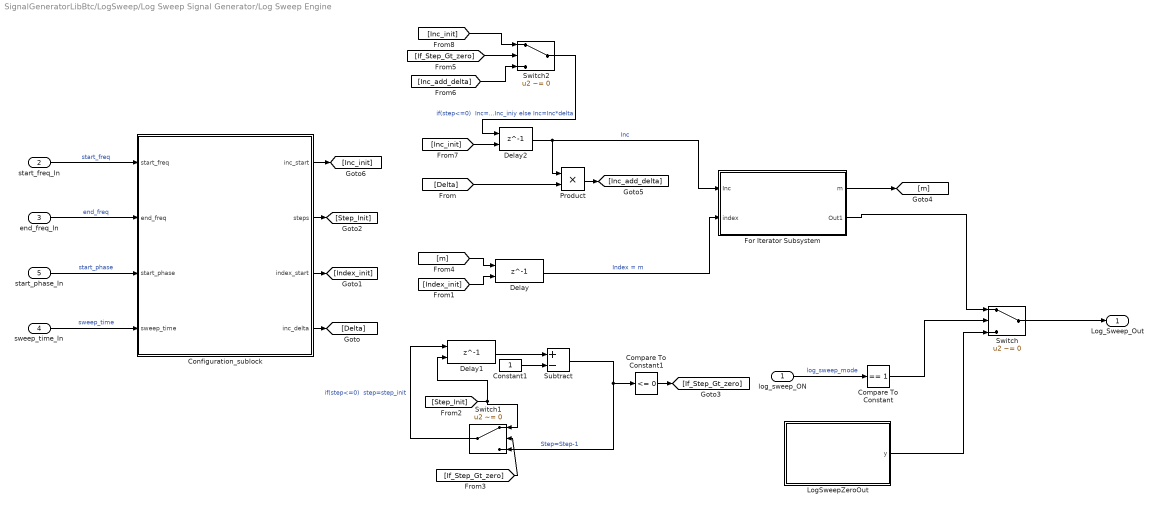
== system SignalGeneratorLibBtc/LogSweep/Log Sweep Signal Generator/Log Sweep Engine ==
  log_sweep_ON : Inport
  start_freq_In : Inport  Port=2
  end_freq_In : Inport  Port=3
  sweep_time_In : Inport  Port=4
  start_phase_In : Inport  Port=5
  Compare To Constant : simulink/Logic and Bit Operations/Compare To Constant  relop===  const=1  OutDataTypeStr=boolean
  Compare To Constant1 : simulink/Logic and Bit Operations/Compare To Constant  relop=<=  const=0  OutDataTypeStr=boolean
  Configuration_sublock : Subsystem
  Constant1 : Constant  OutDataTypeStr=single
  Delay : Delay  DelayLength=1  InitialConditionSource=Input port
      settings: InputPortMap=u0,p4
  Delay1 : Delay  DelayLength=1  InitialConditionSource=Input port
      settings: InputPortMap=u0,p4
  Delay2 : Delay  DelayLength=1  InitialConditionSource=Input port
      settings: InputPortMap=u0,p4
  For Iterator Subsystem : Subsystem  TreatAsAtomicUnit=on
  LogSweepZeroOut : MATLAB Function  TreatAsAtomicUnit=on  mask{Nch=Config.NumChannel, frameSize_samples=Config.FrameSizeSamples}
  Product : Product
  Subtract : Sum  Inputs=+-
  Switch : Switch  Criteria=u2 ~= 0  SaturateOnIntegerOverflow=off  InputSameDT=off
  Switch1 : Switch  Criteria=u2 ~= 0  SaturateOnIntegerOverflow=off  InputSameDT=off
  Switch2 : Switch  Criteria=u2 ~= 0  SaturateOnIntegerOverflow=off  InputSameDT=off
  Log_Sweep_Out : Outport  VectorParamsAs1DForOutWhenUnconnected=off
  wires:
  LogSweepZeroOut/1(y) -> Switch/3
  Switch2/1 -> Delay2/1  "if(step<=0)  Inc=Inc_iniy else Inc=Inc*delta"
  [Inc_init] -> Switch2/1
  [Inc_init] -> Delay2/2
  [Inc_add_delta] -> Switch2/3
  Product/1 -> [Inc_add_delta]
  [If_Step_Gt_zero] -> Switch2/2
  [Delta] -> Product/2
  [m] -> Delay/1
  [If_Step_Gt_zero] -> Switch1/2
  Compare To Constant1/1 -> [If_Step_Gt_zero]
  [Step_Init] -> Switch1/1, Delay1/2
  [Index_init] -> Delay/2
  Configuration_sublock/3(index_start) -> [Index_init]
  Delay2/1 -> Product/1, For Iterator Subsystem/1("Inc ")  "Inc"
  Switch1/1 -> Delay1/1  "if(step<=0)  step=step_init"
  Delay1/1 -> Subtract/1
  Constant1/1 -> Subtract/2
  Subtract/1 -> Compare To Constant1/1, Switch1/3  "Step=Step-1"
  Delay/1 -> For Iterator Subsystem/2(index)  "Index = m"
  For Iterator Subsystem/1(m) -> [m]
  For Iterator Subsystem/2(Out1) -> Switch/1
  Configuration_sublock/2(steps) -> [Step_Init]
  Configuration_sublock/4(inc_delta) -> [Delta]
  Configuration_sublock/1(inc_start) -> [Inc_init]
  Switch/1 -> Log_Sweep_Out/1
  Compare To Constant/1 -> Switch/2
  log_sweep_ON/1 -> Compare To Constant/1  "log_sweep_mode"
  sweep_time_In/1 -> Configuration_sublock/4("sweep_time ")  "sweep_time"
  start_phase_In/1 -> Configuration_sublock/3(start_phase)  "start_phase"
  end_freq_In/1 -> Configuration_sublock/2(end_freq)  "end_freq"
  start_freq_In/1 -> Configuration_sublock/1(start_freq)  "start_freq"

== system SignalGeneratorLibBtc/LogSweep/Log Sweep Signal Generator/SimulationTimeTriggered_Subsystem ==
  Constant : Constant
  Digital Clock : DigitalClock  SampleTime=-1
  Equal : RelationalOperator  Operator===  OutDataTypeStr=boolean  RndMeth=Simplest  InputSameDT=off
  SimuliationTimeTriggerdOut1 : Outport  VectorParamsAs1DForOutWhenUnconnected=off
  wires:
  Equal/1 -> SimuliationTimeTriggerdOut1/1
  Constant/1 -> Equal/1
  Digital Clock/1 -> Equal/2

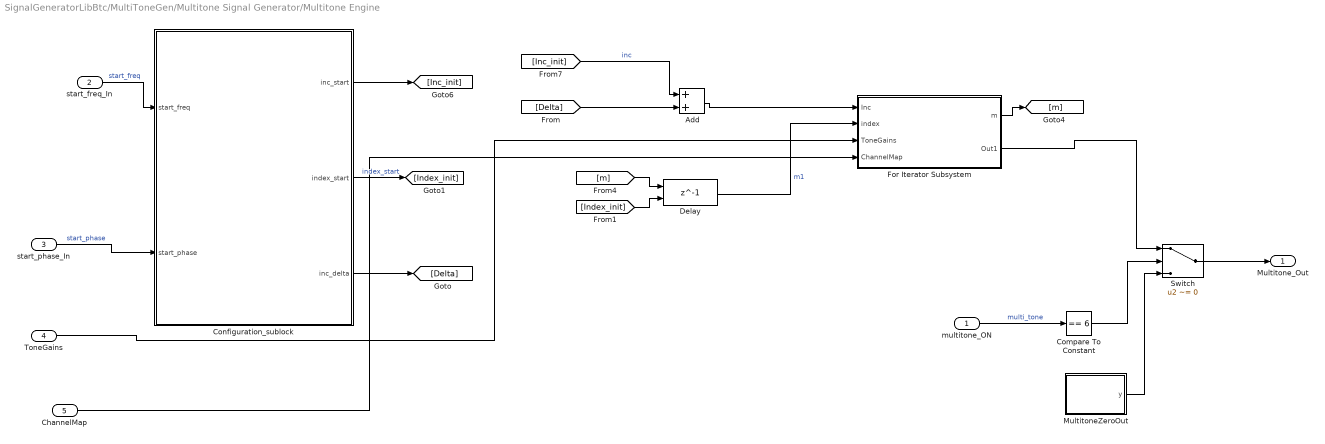
== system SignalGeneratorLibBtc/MultiToneGen/Multitone Signal Generator/Multitone Engine ==
  multitone_ON : Inport
  start_freq_In : Inport  Port=2
  start_phase_In : Inport  Port=3
  ToneGains : Inport  Port=4
  ChannelMap : Inport  Port=5
  Add : Sum
  Compare To Constant : simulink/Logic and Bit Operations/Compare To Constant  relop===  const=6  OutDataTypeStr=boolean
  Configuration_sublock : Subsystem
  Delay : Delay  DelayLength=1  InitialConditionSource=Input port
      settings: InputPortMap=u0,p4
  For Iterator Subsystem : Subsystem  TreatAsAtomicUnit=on
  MultitoneZeroOut : MATLAB Function  TreatAsAtomicUnit=on  mask{frameSize_samples=Config.FrameSizeSamples, Num_Multitone_channels=Config.NumMultitoneChannels}
  Switch : Switch  Criteria=u2 ~= 0  SaturateOnIntegerOverflow=off  InputSameDT=off
  Multitone_Out : Outport  VectorParamsAs1DForOutWhenUnconnected=off
  wires:
  ChannelMap/1 -> For Iterator Subsystem/4(ChannelMap)
  Configuration_sublock/2(index_start) -> [Index_init]  "index_start"
  [Index_init] -> Delay/2
  [m] -> Delay/1
  Delay/1 -> For Iterator Subsystem/2(index)  "m1"
  ToneGains/1 -> For Iterator Subsystem/3(ToneGains)
  [Inc_init] -> Add/1  "inc"
  MultitoneZeroOut/1(y) -> Switch/3
  Add/1 -> For Iterator Subsystem/1("Inc ")
  [Delta] -> Add/2
  For Iterator Subsystem/1(m) -> [m]
  For Iterator Subsystem/2(Out1) -> Switch/1
  Configuration_sublock/3(inc_delta) -> [Delta]
  Configuration_sublock/1(inc_start) -> [Inc_init]
  Switch/1 -> Multitone_Out/1
  Compare To Constant/1 -> Switch/2
  multitone_ON/1 -> Compare To Constant/1  "multi_tone"
  start_phase_In/1 -> Configuration_sublock/2(start_phase)  "start_phase"
  start_freq_In/1 -> Configuration_sublock/1(start_freq)  "start_freq"

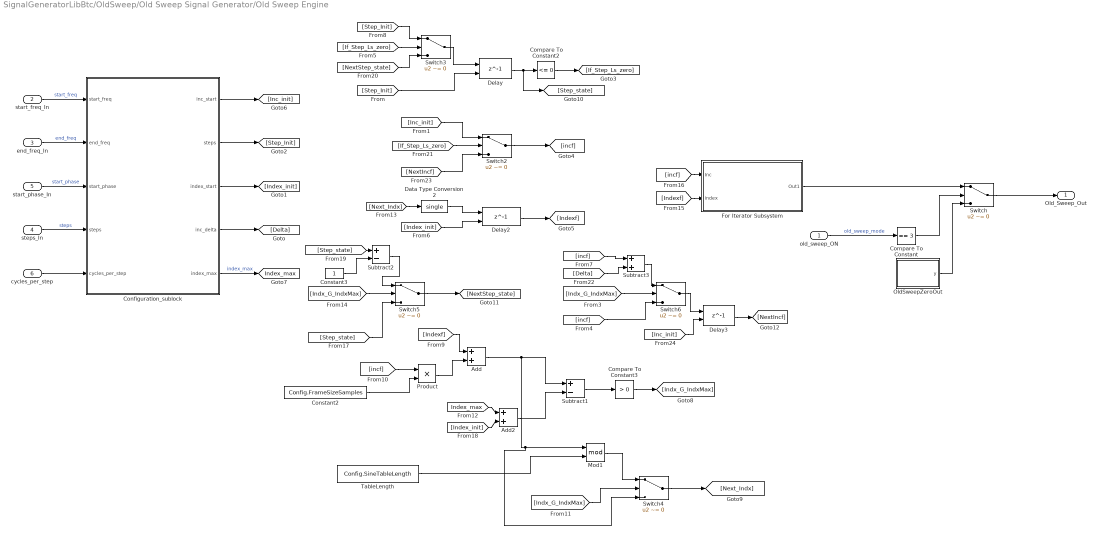
== system SignalGeneratorLibBtc/OldSweep/Old Sweep Signal Generator/Old Sweep Engine ==
  old_sweep_ON : Inport
  start_freq_In : Inport  Port=2
  end_freq_In : Inport  Port=3
  steps_In : Inport  Port=4
  start_phase_In : Inport  Port=5
  cycles_per_step : Inport  Port=6
  Add : Sum
  Add2 : Sum  AccumDataTypeStr=single
  Compare To Constant : simulink/Logic and Bit Operations/Compare To Constant  relop===  const=3  OutDataTypeStr=boolean
  Compare To Constant2 : simulink/Logic and Bit Operations/Compare To Constant  relop=<=  const=0  OutDataTypeStr=boolean
  Compare To Constant3 : simulink/Logic and Bit Operations/Compare To Constant  relop=>  const=0  OutDataTypeStr=boolean
  Configuration_sublock : Subsystem
  Constant2 : Constant  Value=Config.FrameSizeSamples  OutDataTypeStr=uint32
  Constant3 : Constant  OutDataTypeStr=single
  Data Type Conversion2 : DataTypeConversion  OutDataTypeStr=single  SaturateOnIntegerOverflow=off  RndMeth=Floor
  Delay : Delay  DelayLength=1  InitialConditionSource=Input port
      settings: InputPortMap=u0,p4
  Delay2 : Delay  DelayLength=1  InitialConditionSource=Input port
      settings: InputPortMap=u0,p4
  Delay3 : Delay  DelayLength=1  InitialConditionSource=Input port
      settings: InputPortMap=u0,p4
  For Iterator Subsystem : Subsystem  TreatAsAtomicUnit=on
  Mod1 : Math  Operator=mod  SignedPower=on
  OldSweepZeroOut : MATLAB Function  TreatAsAtomicUnit=on  mask{Nch=Config.NumChannel, frameSize_samples=Config.FrameSizeSamples}
  Product : Product
  Subtract1 : Sum  Inputs=+-
  Subtract2 : Sum  Inputs=+-
  Subtract3 : Sum
  Switch{,2..6} (6 alike) : Switch  Criteria=u2 ~= 0  SaturateOnIntegerOverflow=off  InputSameDT=off
  TableLength : Constant  Value=Config.SineTableLength  VectorParams1D=off  OutDataTypeStr=single
  Old_Sweep_Out : Outport  VectorParamsAs1DForOutWhenUnconnected=off
  tag scope: Index_max=global
  wires:
  Data Type Conversion2/1 -> Delay2/1
  Add/1 -> Switch4/3, Mod1/1, Subtract1/1
  TableLength/1 -> Mod1/2
  Delay3/1 -> [NextIncf]
  [Inc_init] -> Delay3/2
  [NextIncf] -> Switch2/3
  Switch6/1 -> Delay3/1
  Subtract3/1 -> Switch6/1
  [Delta] -> Subtract3/2
  [incf] -> Subtract3/1
  [incf] -> Switch6/3
  [Indx_G_IndxMax] -> Switch6/2
  Compare To Constant3/1 -> [Indx_G_IndxMax]
  [NextStep_state] -> Switch3/3
  Switch5/1 -> [NextStep_state]
  Subtract2/1 -> Switch5/1
  Constant3/1 -> Subtract2/2
  [Step_state] -> Subtract2/1
  [Step_state] -> Switch5/3
  [Indx_G_IndxMax] -> Switch5/2
  [Next_Indx] -> Data Type Conversion2/1
  Switch4/1 -> [Next_Indx]
  Mod1/1 -> Switch4/1
  [Indx_G_IndxMax] -> Switch4/2
  Subtract1/1 -> Compare To Constant3/1
  Add2/1 -> Subtract1/2
  [Index_max] -> Add2/1
  [Index_init] -> Add2/2
  Product/1 -> Add/2
  Constant2/1 -> Product/2
  [incf] -> Product/1
  [Indexf] -> Add/1
  Switch3/1 -> Delay/1
  [Step_Init] -> Switch3/1
  [If_Step_Ls_zero] -> Switch3/2
  [Index_init] -> Delay2/2
  Delay2/1 -> [Indexf]
  Switch2/1 -> [incf]
  [Inc_init] -> Switch2/1
  [If_Step_Ls_zero] -> Switch2/2
  Compare To Constant2/1 -> [If_Step_Ls_zero]
  Delay/1 -> [Step_state], Compare To Constant2/1
  [Step_Init] -> Delay/2
  Configuration_sublock/5(index_max) -> [Index_max]  "index_max"
  [incf] -> For Iterator Subsystem/1("Inc ")
  [Indexf] -> For Iterator Subsystem/2(index)
  cycles_per_step/1 -> Configuration_sublock/5(cycles_per_step)
  OldSweepZeroOut/1(y) -> Switch/3
  Configuration_sublock/3(index_start) -> [Index_init]
  For Iterator Subsystem/1(Out1) -> Switch/1
  Configuration_sublock/2(steps) -> [Step_Init]
  Configuration_sublock/4(inc_delta) -> [Delta]
  Configuration_sublock/1(inc_start) -> [Inc_init]
  Switch/1 -> Old_Sweep_Out/1
  Compare To Constant/1 -> Switch/2
  old_sweep_ON/1 -> Compare To Constant/1  "old_sweep_mode"
  steps_In/1 -> Configuration_sublock/4("steps ")  "steps"
  start_phase_In/1 -> Configuration_sublock/3(start_phase)  "start_phase"
  end_freq_In/1 -> Configuration_sublock/2(end_freq)  "end_freq"
  start_freq_In/1 -> Configuration_sublock/1(start_freq)  "start_freq"

== system SignalGeneratorLibBtc/OldSweep/Old Sweep Signal Generator/SimulationTimeTriggered_Subsystem ==
  Constant : Constant  Value=5
  Digital Clock : DigitalClock  SampleTime=-1
  Equal : RelationalOperator  Operator===  OutDataTypeStr=boolean  RndMeth=Simplest  InputSameDT=off
  SimuliationTimeTriggerdOut1 : Outport  VectorParamsAs1DForOutWhenUnconnected=off
  wires:
  Equal/1 -> SimuliationTimeTriggerdOut1/1
  Constant/1 -> Equal/1
  Digital Clock/1 -> Equal/2

== system SignalGeneratorLibBtc/Sawtooth/SawtoothGenSubsystem/SimulationTimeTriggered_Subsystem ==
  Constant : Constant  OutDataTypeStr=single
  Digital Clock : DigitalClock  SampleTime=-1
  Equal : RelationalOperator  Operator===  OutDataTypeStr=boolean  RndMeth=Simplest  InputSameDT=off
  SimuliationTimeTriggerdOut1 : Outport  VectorParamsAs1DForOutWhenUnconnected=off
  wires:
  Equal/1 -> SimuliationTimeTriggerdOut1/1
  Constant/1 -> Equal/1
  Digital Clock/1 -> Equal/2

== system SignalGeneratorLibBtc/Sawtooth/SawtoothGenSubsystem/Subsystem ==
  In1 : Inport
  In2 : Inport  Port=2
  In3 : Inport  Port=3
  Disable_Sawtooth : Subsystem  TreatAsAtomicUnit=on
  If_mode_selection : If  IfExpression=(u1==5)
  Merge : Merge
  SigGen_Sawtooth : Subsystem  TreatAsAtomicUnit=on
  sawtooth_output : Outport  VectorParamsAs1DForOutWhenUnconnected=off
  wires:
  If_mode_selection/1 -> SigGen_Sawtooth/Action
  SigGen_Sawtooth/1(Output1) -> Merge/1  "sawtooth_output"
  In3/1 -> SigGen_Sawtooth/2(start_phase)
  In1/1 -> If_mode_selection/1
  In2/1 -> SigGen_Sawtooth/1(StartFreq)
  If_mode_selection/2 -> Disable_Sawtooth/Action
  Disable_Sawtooth/1(Output) -> Merge/2  "disable_sawtooth_output"
  Merge/1 -> sawtooth_output/1

== system SignalGeneratorLibBtc/WhiteNoiseGen/ForEachSubsystem/Disable_Noise ==
  Action Port : ActionPort
  RandomNoiseZeroOut : MATLAB Function  TreatAsAtomicUnit=on  mask{Nch=Config.NumChannel, frameSize_samples=Config.FrameSizeSamples}
  Output : Outport  VectorParamsAs1DForOutWhenUnconnected=off
  wires:
  RandomNoiseZeroOut/1(y) -> Output/1

== system SignalGeneratorLibBtc/WhiteNoiseGen/ForEachSubsystem/SigGen_Noise ==
  randomnoise : Inport
  Action Port : ActionPort
  For Iterator Subsystem : Subsystem  TreatAsAtomicUnit=on
  noiseOut1 : Outport  VectorParamsAs1DForOutWhenUnconnected=off
  wires:
  For Iterator Subsystem/1(noiseOut1) -> noiseOut1/1
  randomnoise/1 -> For Iterator Subsystem/1(InitSeed)
